simulink model "CM640A_MotAg1Meas"  (R2013b)
settings: Solver=FixedStepDiscrete  SolverMode=SingleTasking  StartTime=0.0  StopTime=1  FixedStep=0.0000625  RelTol=1e-3
undefined symbols (not defined in the file): ARCHGLBPRM_2PI_ULS_F32, COEFFTBLELMSIZE_CNT_U08, COEFFTBLSIZE_CNT_U08, CORRNTBLAGSTEPSIZE_MATRAD_F32, CORRNTBLSIDXOFFS_CNT_U16, CORRNTBLSIZE_CNT_U16, CORRNTBLSIZEMASK_CNT_U08, MOTAG1OFFS_MOTREV_U0P16, MotAg1PrtclFlt, MOTAG1PRTCLFLTFAILSTEP_CNT_U16, MOTAG1PRTCLFLTPASSSTEP_CNT_U16, MOTAGDELTAPERCORRNPT_CNT_U16, MOTAGIDXMASK_CNT_U16, MotCtrlMotAg1ErrReg, NtcSts1, sigbuilder_block, SNSRAGMASK_CNT_U32, SNSRERRMASK_CNT_U32, SNSRERRNTCMASK_CNT_U08, SNSRVLTGFLTMASK_CNT_U32, SPIPARMASK_CNT_U32
libraries: simulink x28, FloatToFixd x1, NxtrMax x1, NxtrLim x1
(part 4 of 4)

== system CM640A_MotAg1Meas/MotAg1Meas/MotAg1MeasInit1/Compute Correction Table/NVM Ok/Calculate Correction Table/Change Correction Coordinate/Waveform Coordinate Change/Determine Non Wrapped Correction Term/Calculate Correction Term1/Calculate Correction Term ==
  Y1 : Inport
  Y2 : Inport  Port=2
  IndexScale : Inport  Port=3
  ReconstructedWaveform[x] : Inport  Port=4
  ReconstructedWaveform[x+1] : Inport  Port=5
  Action Port : ActionPort  ActionType=else
  CopyRight2 : Subsystem  Description=|  mask(Copyright Information){none=on}
      | Copyright info block.                                               
      |                                                                     
      | Place copyright information at the top of every subsystem in design.
      mask prompts: none "No parameters"
      mask help: Place copyright information at the top of every subsystem in design.
      mask Display:
      | NxtrConf = 'Nexteer Confidential';
      | 
      | sys = bdroot; %handle for the current model ("system")
      | first = get_param(sys,'Created');
      | first = first(end-3:end);  %year is last four digits
      | 
      | last = get_param(sys,'LastModifiedDate');
      | if isempty(last)
      |     last = datestr(now,'yyyy');
      | else
      |     last = last(end-3:end);
      | end
      | 
      | if strcmp(first,last)
      |     fprintf('%s -- Copyright %s Nexteer',NxtrConf,first)
      | else
      |     fprintf('%s -- %s%s- %s Nexteer',NxtrConf,char(169),first,last)
      | end
  Divide : Product  Inputs=*/
  Product : Product
  Subtract : Sum  Inputs=+-
  Subtract1 : Sum  Inputs=+-
  Subtract2 : Sum  Inputs=+-
  Subtract3 : Sum
  CorrnTerm_Found : Outport
  wires:
  IndexScale/1 -> Subtract1/1
  Y2/1 -> Subtract/1
  Y1/1 -> Subtract1/2, Subtract/2
  Subtract1/1 -> Divide/1
  Subtract/1 -> Divide/2
  Divide/1 -> Product/1
  ReconstructedWaveform[x+1]/1 -> Subtract2/1
  ReconstructedWaveform[x]/1 -> Subtract2/2, Subtract3/2
  Subtract2/1 -> Product/2
  Product/1 -> Subtract3/1
  Subtract3/1 -> CorrnTerm_Found/1

== system CM640A_MotAg1Meas/MotAg1Meas/MotAg1MeasInit1/Compute Correction Table/NVM Ok/Calculate Correction Table/Change Correction Coordinate/Waveform Coordinate Change/Determine Non Wrapped Correction Term/Calculate Correction Term1/CopyRight2 ==

== system CM640A_MotAg1Meas/MotAg1Meas/MotAg1MeasInit1/Compute Correction Table/NVM Ok/Calculate Correction Table/Change Correction Coordinate/Waveform Coordinate Change/Determine Non Wrapped Correction Term/Calculate Correction Term1/Denominator == 0 ==
  Action Port : ActionPort  ActionType=then
  Constant : Constant  Value=0  OutDataTypeStr=single
  CopyRight2 : Subsystem  Description=|  mask(Copyright Information){none=on}
      | Copyright info block.                                               
      |                                                                     
      | Place copyright information at the top of every subsystem in design.
      mask prompts: none "No parameters"
      mask help: Place copyright information at the top of every subsystem in design.
      mask Display:
      | NxtrConf = 'Nexteer Confidential';
      | 
      | sys = bdroot; %handle for the current model ("system")
      | first = get_param(sys,'Created');
      | first = first(end-3:end);  %year is last four digits
      | 
      | last = get_param(sys,'LastModifiedDate');
      | if isempty(last)
      |     last = datestr(now,'yyyy');
      | else
      |     last = last(end-3:end);
      | end
      | 
      | if strcmp(first,last)
      |     fprintf('%s -- Copyright %s Nexteer',NxtrConf,first)
      | else
      |     fprintf('%s -- %s%s- %s Nexteer',NxtrConf,char(169),first,last)
      | end
  CorrTerm Found : Outport
  wires:
  Constant/1 -> CorrTerm Found/1

== system CM640A_MotAg1Meas/MotAg1Meas/MotAg1MeasInit1/Compute Correction Table/NVM Ok/Calculate Correction Table/Build Wave/Reconstructed Waveform Processing/Harmonic Coefficient Processing/SinCos (Use library function from NxtrMath)/Calc Range Limited Cosine - 2 Term/CopyRight2 ==

== system CM640A_MotAg1Meas/MotAg1Meas/MotAg1MeasInit1/Compute Correction Table/NVM Ok/Calculate Correction Table/Build Wave/Reconstructed Waveform Processing/Harmonic Coefficient Processing/SinCos (Use library function from NxtrMath)/Calc Range Limited Sine - 2 Term/CopyRight2 ==

== system CM640A_MotAg1Meas/MotAg1Meas/MotAg1MeasInit1/Compute Correction Table/NVM Ok/Calculate Correction Table/Change Correction Coordinate/Waveform Coordinate Change/Determine Non Wrapped Correction Term/Calculate Correction Term1/Calculate Correction Term/CopyRight2 ==

== system CM640A_MotAg1Meas/MotAg1Meas/MotAg1MeasInit1/Compute Correction Table/NVM Ok/Calculate Correction Table/Change Correction Coordinate/Waveform Coordinate Change/Determine Non Wrapped Correction Term/Calculate Correction Term1/Denominator == 0/CopyRight2 ==

== stateflow chart CM640A_MotAg1Meas/MotAg1Meas/MotAg1MeasPer1/Compensate MechMtrPos/Normalize MechMtrPos1 ==
  (default) -> (junction 2) : {
      | MechMtrPos1_Out = MechMtrPos1_In;
      | }
  (junction 6) -> (junction 2)
  (junction 9) -> (junction 2)
  (junction 2) -> (junction 6) [order 1] : [
      | MechMtrPos1_Out < 0
      | ]
      | {
      | MechMtrPos1_Out = MechMtrPos1_Out + 65536;
      | }
  (junction 2) -> (junction 9) [order 2] : [
      | MechMtrPos1_Out > 65535
      | ]
      | {
      | MechMtrPos1_Out = MechMtrPos1_Out - 65536;
      | }
  (junction 2) -> (junction 26) [order 3]
  (junction 26) -> (junction 12) [order 1] : [
      | MtrPosPolarity_Cnt_s8 < 0
      | ]
      | {
      | MechMtrPos1_Out = 65535 - MechMtrPos1_Out;
      | }
  (junction 26) -> (junction 12) [order 2]
  data: MtrPosPolarity_Cnt_s8 input int8; MechMtrPos1_Out output int32; MechMtrPos1_In input int32

== stateflow chart CM640A_MotAg1Meas/MotAg1Meas/MotAg1MeasPer1/Process MotAg1 Angle/Chart ==
  (default) -> (junction 5)
  (junction 5) -> (junction 7) [order 1] : [Fault != 0]
  (junction 7) -> (junction 10) [order 1] : [FaultCntPrev == 65535]
      | {
      | FaultCnt = 0;
      | }
  (junction 7) -> (junction 10) [order 2] : {
      | FaultCnt = FaultCntPrev+1;
      | }
  (junction 5) -> (junction 8) [order 2] : {
      | FaultCnt = FaultCntPrev;
      | }
  (junction 8) -> (junction 10)
  data: Fault input uint16; FaultCntPrev input uint16; FaultCnt output uint16

== stateflow chart CM640A_MotAg1Meas/MotAg1Meas/MotAg1MeasPer1/Process MotAg1 Angle/Chart1 ==
  (default) -> (junction 5)
  (junction 5) -> (junction 7) [order 1] : [Fault != 0]
  (junction 7) -> (junction 10) [order 1] : [FaultCntPrev == 65535]
      | {
      | FaultCnt = 0;
      | }
  (junction 7) -> (junction 10) [order 2] : {
      | FaultCnt = FaultCntPrev+1;
      | }
  (junction 5) -> (junction 8) [order 2] : {
      | FaultCnt = FaultCntPrev;
      | }
  (junction 8) -> (junction 10)
  data: Fault input uint16; FaultCntPrev input uint16; FaultCnt output uint16

== stateflow chart CM640A_MotAg1Meas/MotAg1Meas/MotAg1MeasPer2/Process ErrorReg and DieRevCtr/Process MotAg1RawErr/Chart1 ==
  (default) -> (junction 5)
  (junction 5) -> (junction 7) [order 1] : [Fault != 0]
  (junction 7) -> (junction 10) [order 1] : [FaultCntPrev == 65535]
      | {
      | FaultCnt = 0;
      | }
  (junction 7) -> (junction 10) [order 2] : {
      | FaultCnt = FaultCntPrev+1;
      | }
  (junction 5) -> (junction 8) [order 2] : {
      | FaultCnt = FaultCntPrev;
      | }
  (junction 8) -> (junction 10)
  data: Fault input uint16; FaultCntPrev input uint16; FaultCnt output uint16

== stateflow chart CM640A_MotAg1Meas/MotAg1Meas/MotAg1MeasPer1/Process MotAg1 Angle/Chart2 ==
  (default) -> (junction 5)
  (junction 5) -> (junction 7) [order 1] : [Delta != 0]
  (junction 7) -> (junction 10) [order 1] : [RollngCntPrev == 255]
      | {
      | RollngCnt = 0;
      | }
  (junction 7) -> (junction 10) [order 2] : {
      | RollngCnt = RollngCntPrev+1;
      | }
  (junction 5) -> (junction 8) [order 2] : {
      | RollngCnt = RollngCntPrev;
      | }
  (junction 8) -> (junction 10)
  data: Delta input uint8; RollngCntPrev input uint8; RollngCnt output uint8

== stateflow chart CM640A_MotAg1Meas/MotAg1Meas/MotAg1MeasPer2/MotAg1 Protocol Fault Operation/SetNtcSts/ISO Fault Debounce Design ==
  note: NTCSTS_PASSD           (0)
      | NTCSTS_FAILD             (1)
      | NTCSTS_PREPASSD   (2)
      | NTCSTS_PREFAILD     (3)
      |
      | SIGQLFR_NORES        (0)
      | SIGQLFR_PASSD         (1)
      | SIGQLFR_FAILD           (2)
  note: Pass Loop
  note: Fail Loop
  note: 
  (default) -> (junction 89)
  (junction 89) -> (junction 95) [order 1] : [NtcSts ==3]
  (junction 89) -> (junction 93) [order 2] : [NtcSts ==2]
  (junction 89) -> (junction 141) [order 3] : [NtcSts ==1]
      | { ErrAcc = 32767;
      | Qualifier =2;
      |  }
  (junction 89) -> (junction 141) [order 4] : [NtcSts ==0]
      | { ErrAcc = -32768;
      | Qualifier=1;
      | }
  (junction 95) -> (junction 103) [order 2]
  (junction 95) -> (junction 111) [order 1] : [ErrAcc <=0]
      | {ErrAcc = DebStep;}
  (junction 93) -> (junction 123) [order 2] : {
      | ErrAcc = ErrAcc - DebStep;
      | }
  (junction 93) -> (junction 123) [order 1] : [(ErrAcc - DebStep) <= -32768]
      | { ErrAcc = -32768;
      | Qualifier=1;
      | }
  (junction 103) -> (junction 111) [order 1] : [(ErrAcc + DebStep) <32767]
      | {ErrAcc = ErrAcc + DebStep;}
  (junction 103) -> (junction 111) [order 2] : {ErrAcc = 32767;
      | Qualifier =2;}
  (junction 123) -> (junction 141)
  (junction 111) -> (junction 141)
  (junction 141) -> (junction 159) [order 2] : {ErrAcc = 0;
      | Qualifier =0;
      | }
  (junction 141) -> (junction 159) [order 1] : [SvcClr ==0]
  data: NtcSts input uint8; Qualifier output uint8; DebStep input uint16; ErrAcc local int16; SvcClr input

== matlab function CM640A_MotAg1Meas/MotAg1Meas/MotAg1MeasInit1/Compute Correction Table/NVM Ok/Calculate Correction Table/Build Wave/Reconstructed Waveform Processing/Harmonic Coefficient Processing/SinCos (Use library function from NxtrMath)/Truth Table ==
  data: RngLimitedSin input; RngLimitedCos input; ThetaIndex input; Sin output; Cos output; SIN225DEG_ULS_F32 input; SIN675DEG_ULS_F32 input; SIN450DEG_ULS_F32 input
function [Sin, Cos] = fcn(RngLimitedSin, RngLimitedCos, ThetaIndex, SIN225DEG_ULS_F32, SIN675DEG_ULS_F32, SIN450DEG_ULS_F32)

aVarTruthTableCondition_1 = false;
aVarTruthTableCondition_2 = false;
aVarTruthTableCondition_3 = false;
aVarTruthTableCondition_4 = false;
aVarTruthTableCondition_5 = false;
aVarTruthTableCondition_6 = false;
aVarTruthTableCondition_7 = false;
aVarTruthTableCondition_8 = false;
aVarTruthTableCondition_9 = false;
aVarTruthTableCondition_10 = false;
aVarTruthTableCondition_11 = false;
aVarTruthTableCondition_12 = false;
aVarTruthTableCondition_13 = false;
aVarTruthTableCondition_14 = false;
aVarTruthTableCondition_15 = false;
aVarTruthTableCondition_16 = false;


% 0      <= Theta < 11.25 &&
% 348.75 <= Theta < 360

aVarTruthTableCondition_1 = logical(ThetaIndex == 0);

% 11.25  <= Theta < 33.75

aVarTruthTableCondition_2 = logical(ThetaIndex == 1);

% 33.75  <= Theta < 56.25

aVarTruthTableCondition_3 = logical(ThetaIndex == 2);

% 56.25  <= Theta < 78.75

aVarTruthTableCondition_4 = logical(ThetaIndex == 3);

% 78.75  <= Theta < 101.25

aVarTruthTableCondition_5 = logical(ThetaIndex == 4);

% 101.25 <= Theta < 123.75

aVarTruthTableCondition_6 = logical(ThetaIndex == 5);

% 123.75 <= Theta < 146.25

aVarTruthTableCondition_7 = logical(ThetaIndex == 6);

% 146.25 <= Theta < 168.75

aVarTruthTableCondition_8 = logical(ThetaIndex == 7);

% 168.75 <= Theta < 191.25

aVarTruthTableCondition_9 = logical(ThetaIndex == 8);

% 191.25 <= Theta < 213.75

aVarTruthTableCondition_10 = logical(ThetaIndex == 9);

% 213.75 <= Theta < 236.25

aVarTruthTableCondition_11 = logical(ThetaIndex == 10);

% 236.25 <= Theta < 258.75

aVarTruthTableCondition_12 = logical(ThetaIndex == 11);

% 258.75 <= Theta < 281.25

aVarTruthTableCondition_13 = logical(ThetaIndex == 12);

% 281.25 <= Theta < 303.75

aVarTruthTableCondition_14 = logical(ThetaIndex == 13);

% 303.75 <= Theta < 326.75

aVarTruthTableCondition_15 = logical(ThetaIndex == 14);

% 326.75 <= Theta < 348.75

aVarTruthTableCondition_16 = logical(ThetaIndex == 15);

if (aVarTruthTableCondition_1)
    aFcnTruthTableAction_1();
elseif (aVarTruthTableCondition_2)
    aFcnTruthTableAction_2();
elseif (aVarTruthTableCondition_3)
    aFcnTruthTableAction_3();
elseif (aVarTruthTableCondition_4)
    aFcnTruthTableAction_4();
elseif (aVarTruthTableCondition_5)
    aFcnTruthTableAction_5();
elseif (aVarTruthTableCondition_6)
    aFcnTruthTableAction_6();
elseif (aVarTruthTableCondition_7)
    aFcnTruthTableAction_7();
elseif (aVarTruthTableCondition_8)
    aFcnTruthTableAction_8();
elseif (aVarTruthTableCondition_9)
    aFcnTruthTableAction_9();
elseif (aVarTruthTableCondition_10)
    aFcnTruthTableAction_10();
elseif (aVarTruthTableCondition_11)
    aFcnTruthTableAction_11();
elseif (aVarTruthTableCondition_12)
    aFcnTruthTableAction_12();
elseif (aVarTruthTableCondition_13)
    aFcnTruthTableAction_13();
elseif (aVarTruthTableCondition_14)
    aFcnTruthTableAction_14();
elseif (aVarTruthTableCondition_15)
    aFcnTruthTableAction_15();
else % Default
    aFcnTruthTableAction_16();
end

function aFcnTruthTableAction_1()

% Example action 1 called from D1 & D2 column in condition table

Sin = RngLimitedSin;
Cos = RngLimitedCos;

function aFcnTruthTableAction_2()


Sin =  SIN675DEG_ULS_F32 * RngLimitedSin + SIN225DEG_ULS_F32 * RngLimitedCos;
Cos = -SIN225DEG_ULS_F32 * RngLimitedSin + SIN675DEG_ULS_F32 * RngLimitedCos;

function aFcnTruthTableAction_3()


Sin =  SIN450DEG_ULS_F32 * RngLimitedSin + SIN450DEG_ULS_F32 * RngLimitedCos;
Cos = -SIN450DEG_ULS_F32 * RngLimitedSin + SIN450DEG_ULS_F32 * RngLimitedCos;

function aFcnTruthTableAction_4()


Sin =  SIN225DEG_ULS_F32 * RngLimitedSin + SIN675DEG_ULS_F32 * RngLimitedCos;
Cos = -SIN675DEG_ULS_F32 * RngLimitedSin + SIN225DEG_ULS_F32 * RngLimitedCos;

function aFcnTruthTableAction_5()


Sin = RngLimitedCos;
Cos = -RngLimitedSin;

function aFcnTruthTableAction_6()


Sin = -SIN225DEG_ULS_F32 * RngLimitedSin + SIN675DEG_ULS_F32 * RngLimitedCos;
Cos = -SIN675DEG_ULS_F32 * RngLimitedSin + -SIN225DEG_ULS_F32 * RngLimitedCos;

function aFcnTruthTableAction_7()


Sin = -SIN450DEG_ULS_F32 * RngLimitedSin + SIN450DEG_ULS_F32 * RngLimitedCos;
Cos = -SIN450DEG_ULS_F32 * RngLimitedSin + -SIN450DEG_ULS_F32 * RngLimitedCos;

function aFcnTruthTableAction_8()


Sin = -SIN675DEG_ULS_F32 * RngLimitedSin + SIN225DEG_ULS_F32 * RngLimitedCos;
Cos = -SIN225DEG_ULS_F32 * RngLimitedSin + -SIN675DEG_ULS_F32 * RngLimitedCos;

function aFcnTruthTableAction_9()


Sin = -RngLimitedSin;
Cos = -RngLimitedCos;

function aFcnTruthTableAction_10()


Sin = -SIN675DEG_ULS_F32 * RngLimitedSin + -SIN225DEG_ULS_F32 * RngLimitedCos;
Cos =  SIN225DEG_ULS_F32 * RngLimitedSin + -SIN675DEG_ULS_F32 * RngLimitedCos;

function aFcnTruthTableAction_11()


Sin = -SIN450DEG_ULS_F32 * RngLimitedSin + -SIN450DEG_ULS_F32 * RngLimitedCos;
Cos =  SIN450DEG_ULS_F32 * RngLimitedSin + -SIN450DEG_ULS_F32 * RngLimitedCos;

function aFcnTruthTableAction_12()


Sin = -SIN225DEG_ULS_F32 * RngLimitedSin + -SIN675DEG_ULS_F32 * RngLimitedCos;
Cos =  SIN675DEG_ULS_F32 * RngLimitedSin + -SIN225DEG_ULS_F32 * RngLimitedCos;

function aFcnTruthTableAction_13()


Sin = -RngLimitedCos;
Cos =  RngLimitedSin;

function aFcnTruthTableAction_14()


Sin =  SIN225DEG_ULS_F32 * RngLimitedSin + -SIN675DEG_ULS_F32 * RngLimitedCos;
Cos =  SIN675DEG_ULS_F32 * RngLimitedSin +  SIN225DEG_ULS_F32 * RngLimitedCos;

function aFcnTruthTableAction_15()


Sin =  SIN450DEG_ULS_F32 * RngLimitedSin + -SIN450DEG_ULS_F32 * RngLimitedCos;
Cos =  SIN450DEG_ULS_F32 * RngLimitedSin +  SIN450DEG_ULS_F32 * RngLimitedCos;

function aFcnTruthTableAction_16()

% Example action 2 called from D3 column in condition table

Sin =  SIN675DEG_ULS_F32 * RngLimitedSin + -SIN225DEG_ULS_F32 * RngLimitedCos;
Cos =  SIN225DEG_ULS_F32 * RngLimitedSin +  SIN675DEG_ULS_F32 * RngLimitedCos;

== matlab function CM640A_MotAg1Meas/MotAg1Meas/MotAg1MeasInit1/Compute Correction Table/NVM Ok/Calculate Correction Table/Change Correction Coordinate/Waveform Coordinate Change/Calculate Index Scale/Truth Table ==
  data: ReconWfrm_0 input; IndexScale output single; LoopIndex input; ARCHGLBPRM_2PI_ULS_F32 input
function IndexScale = fcn(ReconWfrm_0, LoopIndex, ARCHGLBPRM_2PI_ULS_F32)

aVarTruthTableCondition_1 = false;
aVarTruthTableCondition_2 = false;
aVarTruthTableCondition_3 = false;


% First entry in reconstructed waveform is >= 0

aVarTruthTableCondition_1 = logical(ReconWfrm_0 >= 0);

% Reconstructed waveform is positively wrapped around

aVarTruthTableCondition_2 = logical(ReconWfrm_0 > LoopIndex);

% Reconstructed waveform is negatively wrapped around

aVarTruthTableCondition_3 = logical((ReconWfrm_0 + ARCHGLBPRM_2PI_ULS_F32) <= LoopIndex);

if (aVarTruthTableCondition_1 && aVarTruthTableCondition_2)
    aFcnTruthTableAction_1();
elseif (aVarTruthTableCondition_1)
    aFcnTruthTableAction_3();
elseif (aVarTruthTableCondition_3)
    aFcnTruthTableAction_2();
else % Default
    aFcnTruthTableAction_3();
end

function aFcnTruthTableAction_1()

% Reconstructed waveform is positively wrapped around - add 2pi for alignment

IndexScale = LoopIndex + ARCHGLBPRM_2PI_ULS_F32;

function aFcnTruthTableAction_2()

% Reconstructed waveform is negatively wrapped around - subtract 2pi for alignment

IndexScale = LoopIndex - ARCHGLBPRM_2PI_ULS_F32;

function aFcnTruthTableAction_3()

% Reconstructed waveform and loop index are not wrapped relative to one another

IndexScale = LoopIndex;
